simulink model "F500Heli_PIDAttidudeInTheBackLoop"  (R2022b)
settings: Solver=ode3  StartTime=0.0  StopTime=80  FixedStep=0.01  RelTol=1e-3  EnableMultiTasking=on
libraries: simulink_need_slupdate x15, simulink x5
settings Model: Creator=zhi  LastModifiedBy=henrr
settings SolverCC: AlgebraicLoopSolver=TrustRegion
settings DataIOCC: LimitDataPoints=on  SaveFormat=Array  SignalLoggingSaveFormat=ModelDataLogs  ReturnWorkspaceOutputs=off
settings OptimizationCC: ExpressionDepthLimit=2147483647  LifeSpan=inf
settings DebuggingCC: UnderspecifiedInitializationDetection=Classic  MergeDetectMultiDrivingBlocksExec=none  SolverPrmCheckMsg=warning  FcnCallInpInsideContextMsg=warning  UnconnectedInputMsg=warning  UnconnectedOutputMsg=warning  UnconnectedLineMsg=warning  StateNameClashWarn=warning  SFUnexpectedBacktrackingDiag=warning  SFNoUnconditionalDefaultTransitionDiag=warning  SFExecutionAtInitializationDiag=none  SFMachineParentedDataDiag=warning  ArithmeticOperatorsInVariantConditions=warning
settings HardwareCC: ProdBitPerPointer=32  ProdBitPerSizeT=32  ProdBitPerPtrDiffT=32  ProdLargestAtomicFloat=None  ProdIntDivRoundTo=Undefined  ProdEndianess=Unspecified  ProdWordSize=32  ProdHWDeviceType=32-bit Generic
settings ModelReferenceCC: PropagateSignalLabelsOutOfModel=off
settings SFSimCC: SimUseLocalCustomCode=off  SimParseCustomCode=off  CustomCodeUndefinedFunction=UseInterfaceOnly
settings RTWCC: RTWUseLocalCustomCode=off
settings CodeAppCC: StateflowObjectComments=on
settings GRTTargetCC: TargetLangStandard=C89/C90 (ANSI)  CombineOutputUpdateFcns=off  GRTInterface=on
settings ConfigComp: CovMetricSettings=dw  CovSaveCumulativeToWorkspaceVar=on  CovSaveSingleToWorkspaceVar=on  CovExternalEMLEnable=off

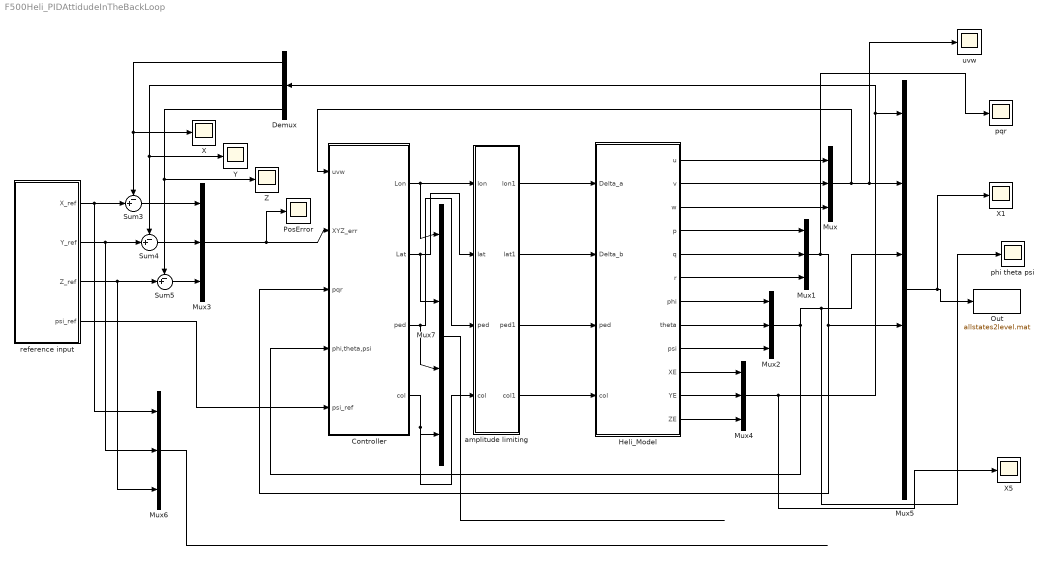
== system F500Heli_PIDAttidudeInTheBackLoop ==
  Controller : Subsystem
  Demux : Demux  Outputs=3
  Heli_Model : Subsystem
  Mux{,1..4,6} (6 alike) : Mux  Inputs=3
  Mux5 : Mux  Inputs=6
  Mux7 : Mux
  Out : ToFile  Filename=allstates2level.mat  MatrixName=AllStates
  PosError : Scope
  Sum3 : Sum  Inputs=-+|
  Sum4 : Sum  Inputs=-+|
  Sum5 : Sum  Inputs=-+|
  X : Scope
  X1 : Scope
  X5 : Scope
  Y : Scope
  Z : Scope
  amplitude limiting : Subsystem
  phi theta psi : Scope
  pqr : Scope
  reference input : Subsystem
  uvw : Scope
  wires:
  Heli_Model/1(u) -> Mux/1
  Heli_Model/2(v) -> Mux/2
  Heli_Model/3(w) -> Mux/3
  Heli_Model/4(p) -> Mux1/1
  Heli_Model/5(q) -> Mux1/2
  Heli_Model/6(r) -> Mux1/3
  Heli_Model/7(phi) -> Mux2/1
  Heli_Model/8(theta) -> Mux2/2
  Heli_Model/9(psi) -> Mux2/3
  Heli_Model/10(XE) -> Mux4/1
  Heli_Model/11(YE) -> Mux4/2
  Heli_Model/12(ZE) -> Mux4/3
  Mux4/1 -> X5/1, Demux/1, Mux5/1
  Mux/1 -> Controller/1(uvw), uvw/1, Mux5/2
  Mux2/1 -> Controller/4(phi,theta,psi), phi theta psi/1, Mux5/3
  Mux1/1 -> pqr/1, Controller/3(pqr), Mux5/4
  Demux/2 -> Sum4/1, Y/1
  Demux/3 -> Sum5/1, Z/1
  reference input/2(Y_ref) -> Sum4/2, Mux6/2
  reference input/3(Z_ref) -> Sum5/2, Mux6/3
  Sum5/1 -> Mux3/3
  Sum4/1 -> Mux3/2
  reference input/1(X_ref) -> Sum3/2, Mux6/1
  Demux/1 -> Sum3/1, X/1
  Sum3/1 -> Mux3/1
  Controller/1(Lon) -> amplitude limiting/1(lon), Mux7/1
  Controller/2(Lat) -> amplitude limiting/2(lat), Mux7/2
  Controller/3(ped) -> amplitude limiting/3(ped), Mux7/3
  Controller/4(col) -> amplitude limiting/4(col), Mux7/4
  amplitude limiting/1(lon1) -> Heli_Model/1(Delta_a)
  amplitude limiting/2(lat1) -> Heli_Model/2(Delta_b)
  amplitude limiting/3(ped1) -> Heli_Model/3(ped)
  amplitude limiting/4(col1) -> Heli_Model/4(col)
  reference input/4(psi_ref) -> Controller/5(psi_ref)
  Mux3/1 -> Controller/2(XYZ_err), PosError/1
  Mux5/1 -> X1/1, Out/1
  Mux7/1 -> ?
  Mux6/1 -> ?

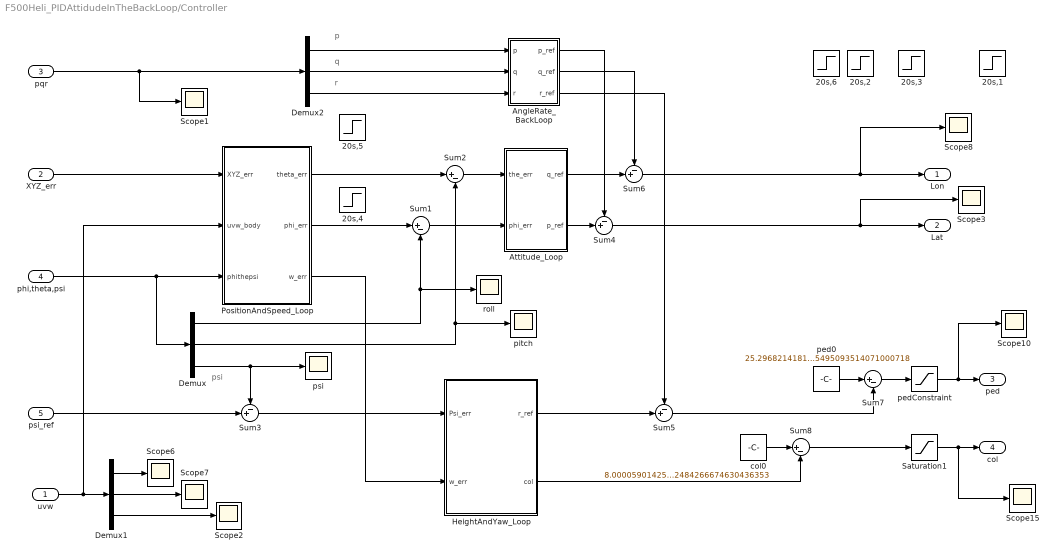
== system F500Heli_PIDAttidudeInTheBackLoop/Controller ==
  note: p
  note: q
  note: r
  note: psi
  uvw : Inport
  XYZ_err : Inport  Port=2
  pqr : Inport  Port=3
  phi,theta,psi : Inport  Port=4
  psi_ref : Inport  Port=5
  20s,1 : Step  Time=0  SampleTime=0
  20s,2 : Step  Time=0  After=0  SampleTime=0
  20s,3 : Step  Time=0  After=25.296753501  SampleTime=0
  20s,4 : Step  Time=0  After=0.2  SampleTime=0
  20s,5 : Step  After=-0.1  SampleTime=0
  20s,6 : Step  Time=0  After=0  SampleTime=0
  AngleRate_BackLoop : Subsystem
  Attitude_Loop : Subsystem
  Demux : Demux  Outputs=3
  Demux1 : Demux  Outputs=3
  Demux2 : Demux  Outputs=3
  HeightAndYaw_Loop : Subsystem
  PositionAndSpeed_Loop : Subsystem
  Saturation1 : Saturate  UpperLimit=12  LowerLimit=0.5
  Scope{1..3,6..8,10,15} (8 alike) : Scope
  Sum{1..2,7..8} (4 alike) : Sum  Inputs=|+-
  Sum{3..6} (4 alike) : Sum  Inputs=-+|
  col0 : Constant  Value=8.0000590142582484266674630436353
  ped0 : Constant  Value=25.296821418115495093514071000718
  pedConstraint : Saturate  UpperLimit=35  LowerLimit=18.7232
  pitch : Scope
  psi : Scope
  roll : Scope
  Lon : Outport
  Lat : Outport  Port=2
  ped : Outport  Port=3
  col : Outport  Port=4
  wires:
  uvw/1 -> Demux1/1, PositionAndSpeed_Loop/2(uvw_body)
  XYZ_err/1 -> PositionAndSpeed_Loop/1(XYZ_err)
  Demux/3 -> Sum3/1, psi/1
  pqr/1 -> Demux2/1, Scope1/1
  Sum3/1 -> HeightAndYaw_Loop/1(Psi_err)
  Demux/1 -> Sum1/2, roll/1
  Demux/2 -> Sum2/2, pitch/1
  Sum2/1 -> Attitude_Loop/1(the_err)
  Sum1/1 -> Attitude_Loop/2(phi_err)
  psi_ref/1 -> Sum3/2
  HeightAndYaw_Loop/1(r_ref) -> Sum5/2
  phi,theta,psi/1 -> Demux/1, PositionAndSpeed_Loop/3(phithepsi)
  Attitude_Loop/2(p_ref) -> Sum4/2
  Attitude_Loop/1(q_ref) -> Sum6/2
  Demux1/3 -> Scope2/1
  Demux1/2 -> Scope7/1
  Demux1/1 -> Scope6/1
  Demux2/2 -> AngleRate_BackLoop/2(q)
  Demux2/1 -> AngleRate_BackLoop/1(p)
  AngleRate_BackLoop/1(p_ref) -> Sum4/1
  AngleRate_BackLoop/2(q_ref) -> Sum6/1
  ped0/1 -> Sum7/1
  Sum7/1 -> pedConstraint/1
  pedConstraint/1 -> ped/1, Scope10/1
  Demux2/3 -> AngleRate_BackLoop/3(r)
  AngleRate_BackLoop/3(r_ref) -> Sum5/1
  col0/1 -> Sum8/1
  Sum8/1 -> Saturation1/1
  Saturation1/1 -> col/1, Scope15/1
  PositionAndSpeed_Loop/3(w_err) -> HeightAndYaw_Loop/2(w_err)
  Sum6/1 -> Lon/1, Scope8/1
  Sum4/1 -> Lat/1, Scope3/1
  Sum5/1 -> Sum7/2
  HeightAndYaw_Loop/2(col) -> Sum8/2
  PositionAndSpeed_Loop/2(phi_err) -> Sum1/1
  PositionAndSpeed_Loop/1(theta_err) -> Sum2/1

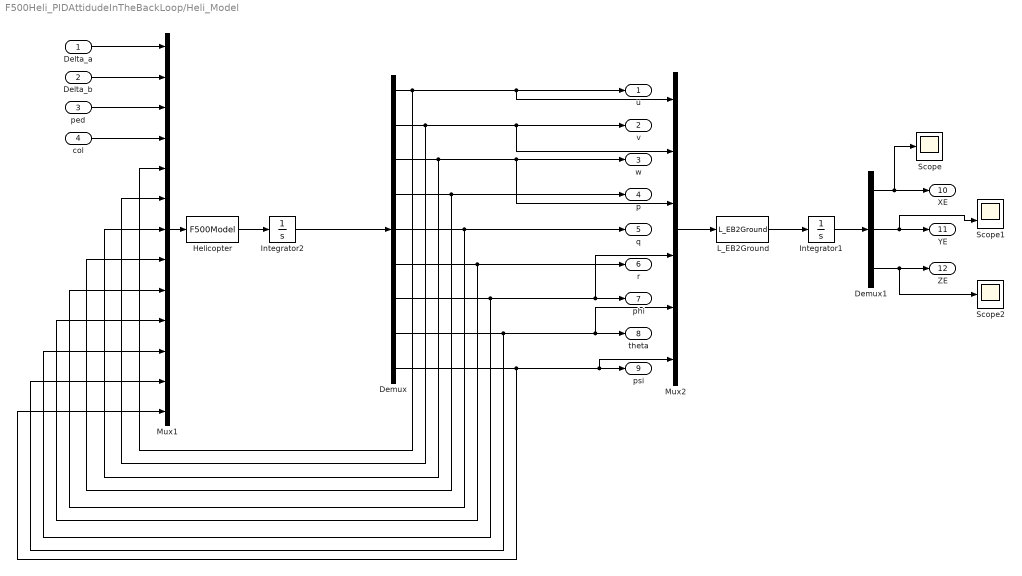
== system F500Heli_PIDAttidudeInTheBackLoop/Heli_Model ==
  Delta_a : Inport
  Delta_b : Inport  Port=2
  ped : Inport  Port=3
  col : Inport  Port=4
  Demux : Demux  Outputs=9
  Demux1 : Demux  Outputs=3
  Helicopter : MATLABFcn  MATLABFcn=F500Model
  Integrator1 : Integrator  InitialCondition=[0 0 0]
  Integrator2 : Integrator  InitialCondition=[0 0 0 0 0 0 0 0 0]
  L_EB2Ground : MATLABFcn  MATLABFcn=L_EB2Ground
  Mux1 : Mux  Inputs=13
  Mux2 : Mux  Inputs=6
  Scope : Scope
  Scope1 : Scope  NumInputPorts=2
  Scope2 : Scope
  u : Outport
  v : Outport  Port=2
  w : Outport  Port=3
  p : Outport  Port=4
  q : Outport  Port=5
  r : Outport  Port=6
  phi : Outport  Port=7
  theta : Outport  Port=8
  psi : Outport  Port=9
  XE : Outport  Port=10
  YE : Outport  Port=11
  ZE : Outport  Port=12
  wires:
  Demux/1 -> Mux1/5, u/1, Mux2/1
  Demux/2 -> Mux1/6, v/1, Mux2/2
  Demux/3 -> Mux1/7, w/1, Mux2/3
  Demux/4 -> Mux1/8, p/1
  Demux/5 -> Mux1/9, q/1
  Demux/6 -> Mux1/10, r/1
  Demux/7 -> Mux1/11, phi/1, Mux2/4
  Demux/8 -> Mux1/12, theta/1, Mux2/5
  Demux/9 -> Mux1/13, psi/1, Mux2/6
  Demux1/1 -> XE/1, Scope/1
  Demux1/2 -> YE/1, Scope1/2
  Demux1/3 -> ZE/1, Scope2/1
  Mux2/1 -> L_EB2Ground/1
  L_EB2Ground/1 -> Integrator1/1
  Integrator1/1 -> Demux1/1
  Mux1/1 -> Helicopter/1
  col/1 -> Mux1/4
  Integrator2/1 -> Demux/1
  ped/1 -> Mux1/3
  Delta_a/1 -> Mux1/1
  Delta_b/1 -> Mux1/2
  Helicopter/1 -> Integrator2/1

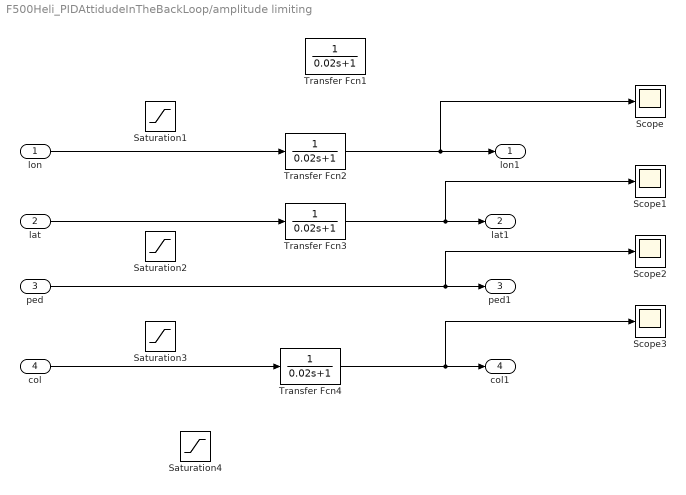
== system F500Heli_PIDAttidudeInTheBackLoop/amplitude limiting ==
  lon : Inport
  lat : Inport  Port=2
  ped : Inport  Port=3
  col : Inport  Port=4
  Saturation1 : Saturate  UpperLimit=0.6  LowerLimit=-0.6
  Saturation2 : Saturate  UpperLimit=0.6  LowerLimit=-0.6
  Saturation3 : Saturate  UpperLimit=0.6  LowerLimit=-0.6
  Saturation4 : Saturate  UpperLimit=10  LowerLimit=-10
  Scope{,1..3} (4 alike) : Scope
  Transfer Fcn{1..4} (4 alike) : TransferFcn  Denominator=[0.02 1]
  lon1 : Outport
  lat1 : Outport  Port=2
  ped1 : Outport  Port=3
  col1 : Outport  Port=4
  wires:
  lon/1 -> Transfer Fcn2/1
  lat/1 -> Transfer Fcn3/1
  col/1 -> Transfer Fcn4/1
  ped/1 -> ped1/1, Scope2/1
  Transfer Fcn2/1 -> lon1/1, Scope/1
  Transfer Fcn3/1 -> lat1/1, Scope1/1
  Transfer Fcn4/1 -> col1/1, Scope3/1

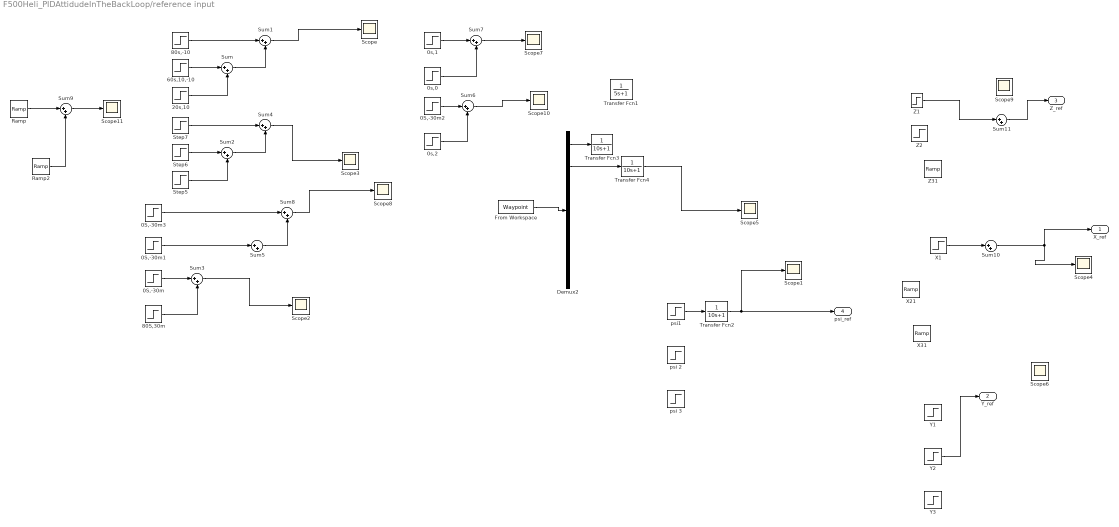
== system F500Heli_PIDAttidudeInTheBackLoop/reference input ==
  0S,-30m : Step  Time=70  After=-3  SampleTime=0
  0S,-30m1 : Step  Time=60  Before=10  After=5  SampleTime=0
  0S,-30m2 : Step  Time=10  After=10  SampleTime=0
  0S,-30m3 : Step  Time=70  Before=5  After=0  SampleTime=0
  0s,0 : Step  Time=10  After=0  SampleTime=0
  0s,1 : Step  Time=0  After=5  SampleTime=0
  0s,2 : Step  Time=0  After=5  SampleTime=0
  20s,10 : Step  Time=20  After=5  SampleTime=0
  60s,10,-10 : Step  Time=30  Before=5  After=-5  SampleTime=0
  80S,30m : Step  Time=10  After=3  SampleTime=0
  80s,-10 : Step  Time=40  Before=-5  After=0  SampleTime=0
  Demux2 : Demux  Outputs=7
  From Workspace : FromWorkspace  VariableName=Waypoint
  Ramp : simulink/Sources/Ramp  slope=1  start=0  InitialOutput=0
  Ramp2 : simulink/Sources/Ramp  slope=-1  start=20  InitialOutput=0
  Scope{,1..11} (12 alike) : Scope
  Step5 : Step  Time=40  After=5  SampleTime=0
  Step6 : Step  Time=50  Before=5  After=-5  SampleTime=0
  Step7 : Step  Time=60  Before=-5  After=0  SampleTime=0
  Sum{,1..11} (12 alike) : Sum  Inputs=|++
  Transfer Fcn1 : TransferFcn  Denominator=[5 1]
  Transfer Fcn2 : TransferFcn  Denominator=[10 1]
  Transfer Fcn3 : TransferFcn  Denominator=[10 1]
  Transfer Fcn4 : TransferFcn  Denominator=[10 1]
  X1 : Step  Time=0  After=20  SampleTime=0
  X21 : simulink/Sources/Ramp  slope=1  start=15  InitialOutput=0
  X31 : simulink/Sources/Ramp  slope=1  start=20  InitialOutput=0
  Y1 : Step  Time=0  After=5  SampleTime=0
  Y2 : Step  Time=0  After=10  SampleTime=0
  Y3 : Step  Time=0  After=5  SampleTime=0
  Z1 : Step  Time=0  After=20  SampleTime=0
  Z2 : Step  Time=10  After=10  SampleTime=0
  Z31 : simulink/Sources/Ramp  slope=1  start=0  InitialOutput=0
  psi 2 : Step  Time=5  After=0.2  SampleTime=0
  psi 3 : Step  Time=0  After=0  SampleTime=0
  psi1 : Step  Time=0  After=0  SampleTime=0
  X_ref : Outport
  Y_ref : Outport  Port=2
  Z_ref : Outport  Port=3
  psi_ref : Outport  Port=4
  wires:
  20s,10/1 -> Sum/2
  60s,10,-10/1 -> Sum/1
  80s,-10/1 -> Sum1/1
  Sum/1 -> Sum1/2
  Sum1/1 -> Scope/1
  Step5/1 -> Sum2/2
  Step6/1 -> Sum2/1
  Step7/1 -> Sum4/1
  Sum2/1 -> Sum4/2
  Sum4/1 -> Scope3/1
  0S,-30m/1 -> Sum3/1
  80S,30m/1 -> Sum3/2
  0S,-30m1/1 -> Sum5/1
  0S,-30m2/1 -> Sum6/1
  0s,2/1 -> Sum6/2
  0s,1/1 -> Sum7/1
  0s,0/1 -> Sum7/2
  Sum8/1 -> Scope8/1
  Sum5/1 -> Sum8/2
  0S,-30m3/1 -> Sum8/1
  Sum3/1 -> Scope2/1
  From Workspace/1 -> Demux2/1
  Demux2/1 -> Transfer Fcn3/1
  Demux2/2 -> Transfer Fcn4/1
  Transfer Fcn2/1 -> psi_ref/1, Scope1/1
  Transfer Fcn4/1 -> Scope5/1
  Sum7/1 -> Scope7/1
  Sum6/1 -> Scope10/1
  Ramp/1 -> Sum9/1
  Sum9/1 -> Scope11/1
  Ramp2/1 -> Sum9/2
  Sum10/1 -> Scope4/1, X_ref/1
  Sum11/1 -> Z_ref/1
  Y2/1 -> Y_ref/1
  psi1/1 -> Transfer Fcn2/1
  Z1/1 -> Sum11/1
  X1/1 -> Sum10/1

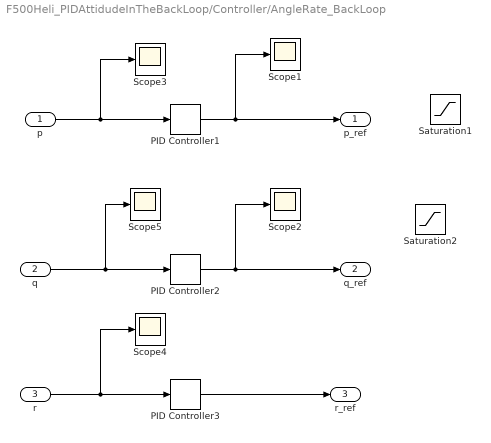
== system F500Heli_PIDAttidudeInTheBackLoop/Controller/AngleRate_BackLoop ==
  p : Inport
  q : Inport  Port=2
  r : Inport  Port=3
  PID Controller1 : simulink_need_slupdate/PID Controller  P=5  I=0  D=0
  PID Controller2 : simulink_need_slupdate/PID Controller  P=5  I=0  D=0
  PID Controller3 : simulink_need_slupdate/PID Controller  P=10  I=0  D=0
  Saturation1 : Saturate  UpperLimit=10  LowerLimit=-10
  Saturation2 : Saturate  UpperLimit=10  LowerLimit=-10
  Scope{1..5} (5 alike) : Scope
  p_ref : Outport
  q_ref : Outport  Port=2
  r_ref : Outport  Port=3
  wires:
  PID Controller1/1 -> Scope1/1, p_ref/1
  p/1 -> PID Controller1/1, Scope3/1
  PID Controller2/1 -> Scope2/1, q_ref/1
  q/1 -> PID Controller2/1, Scope5/1
  r/1 -> PID Controller3/1, Scope4/1
  PID Controller3/1 -> r_ref/1

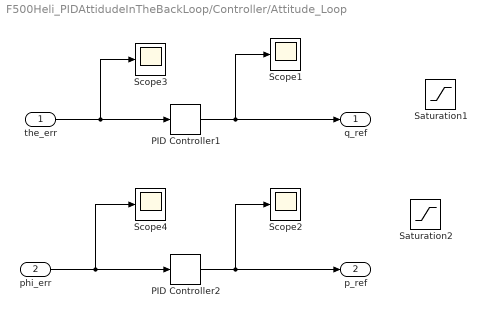
== system F500Heli_PIDAttidudeInTheBackLoop/Controller/Attitude_Loop ==
  the_err : Inport
  phi_err : Inport  Port=2
  PID Controller1 : simulink_need_slupdate/PID Controller  P=20  I=5  D=0
  PID Controller2 : simulink_need_slupdate/PID Controller  P=18  I=5  D=0
  Saturation1 : Saturate  UpperLimit=3  LowerLimit=-3
  Saturation2 : Saturate  UpperLimit=3  LowerLimit=-3
  Scope{1..4} (4 alike) : Scope
  q_ref : Outport
  p_ref : Outport  Port=2
  wires:
  PID Controller1/1 -> Scope1/1, q_ref/1
  the_err/1 -> PID Controller1/1, Scope3/1
  PID Controller2/1 -> Scope2/1, p_ref/1
  phi_err/1 -> PID Controller2/1, Scope4/1

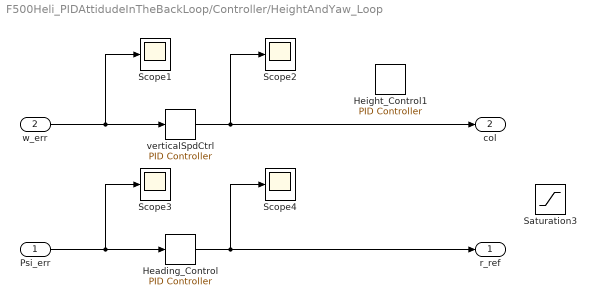
== system F500Heli_PIDAttidudeInTheBackLoop/Controller/HeightAndYaw_Loop ==
  Psi_err : Inport
  w_err : Inport  Port=2
  Heading_Control : simulink_need_slupdate/PID Controller  P=5  I=0  D=0.5
  Height_Control1 : simulink_need_slupdate/PID Controller  P=1  I=0.01  D=1.4
  Saturation3 : Saturate  UpperLimit=36  LowerLimit=18.7232
  Scope{1..4} (4 alike) : Scope
  verticalSpdCtrl : simulink_need_slupdate/PID Controller  P=5  I=0  D=0
  r_ref : Outport
  col : Outport  Port=2
  wires:
  w_err/1 -> verticalSpdCtrl/1, Scope1/1
  verticalSpdCtrl/1 -> Scope2/1, col/1
  Heading_Control/1 -> Scope4/1, r_ref/1
  Psi_err/1 -> Heading_Control/1, Scope3/1

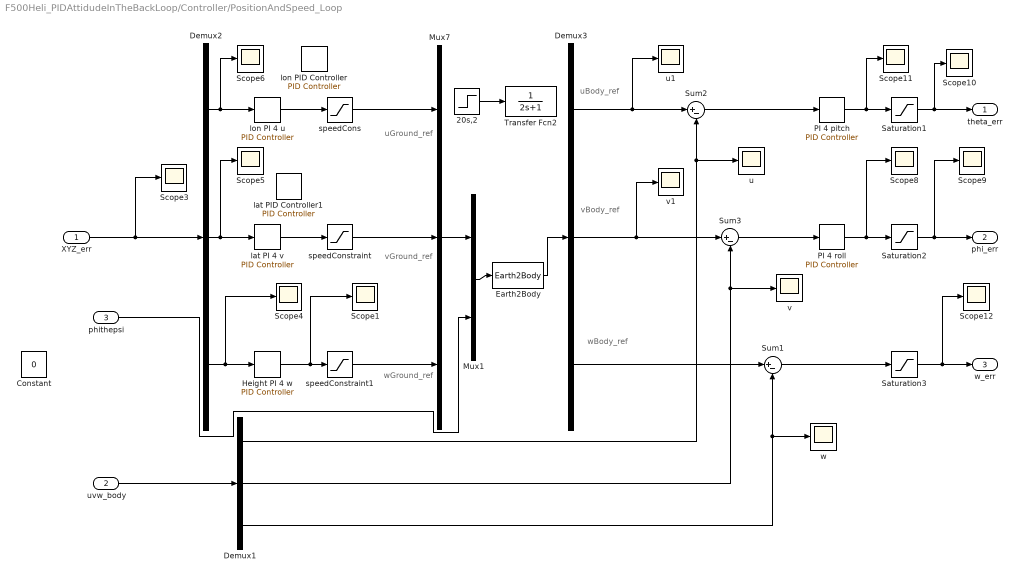
== system F500Heli_PIDAttidudeInTheBackLoop/Controller/PositionAndSpeed_Loop ==
  note: uGround_ref
  note: vGround_ref
  note: wGround_ref
  note: uBody_ref
  note: vBody_ref
  note: wBody_ref
  XYZ_err : Inport
  uvw_body : Inport  Port=2
  phithepsi : Inport  Port=3
  20s,2 : Step  Time=10  After=5  SampleTime=0
  Constant : Constant  Value=0
  Demux1 : Demux  Outputs=3
  Demux2 : Demux  Outputs=3
  Demux3 : Demux  Outputs=3
  Earth2Body : MATLABFcn  MATLABFcn=Earth2Body  OutputDimensions=3
  Height PI 4 w : simulink_need_slupdate/PID Controller  P=1  I=0.002  D=0
  Mux1 : Mux  Inputs=2
  Mux7 : Mux  Inputs=3
  PI 4 pitch : simulink_need_slupdate/PID Controller  P=-0.7  I=0.0001  D=0
  PI 4 roll : simulink_need_slupdate/PID Controller  P=0.7  I=0.0001  D=0
  Saturation1 : Saturate  UpperLimit=0.1745  LowerLimit=-0.5236
  Saturation2 : Saturate  UpperLimit=0.6109  LowerLimit=-0.6109
  Saturation3 : Saturate  UpperLimit=0.6109  LowerLimit=-0.6109
  Scope{1,3..6,8..12} (10 alike) : Scope
  Sum1 : Sum  Inputs=|+-
  Sum2 : Sum  Inputs=|+-
  Sum3 : Sum  Inputs=|+-
  Transfer Fcn2 : TransferFcn  Denominator=[2 1]
  lat PI 4 v : simulink_need_slupdate/PID Controller  P=1  I=0.0001  D=0
  lat PID Controller1 : simulink_need_slupdate/PID Controller  P=1  I=0.0001  D=2
  lon PI 4 u : simulink_need_slupdate/PID Controller  P=1  I=0.0001  D=0
  lon PID Controller : simulink_need_slupdate/PID Controller  P=-1  I=0.0001  D=-2
  speedCons : Saturate  UpperLimit=10  LowerLimit=-10
  speedConstraint : Saturate  UpperLimit=2  LowerLimit=-2
  speedConstraint1 : Saturate  UpperLimit=3  LowerLimit=-3
  u : Scope
  u1 : Scope
  v : Scope
  v1 : Scope
  w : Scope
  theta_err : Outport
  phi_err : Outport  Port=2
  w_err : Outport  Port=3
  wires:
  Demux2/1 -> lon PI 4 u/1, Scope6/1
  lon PI 4 u/1 -> speedCons/1
  lat PI 4 v/1 -> speedConstraint/1
  Demux2/2 -> lat PI 4 v/1, Scope5/1
  Demux2/3 -> Height PI 4 w/1, Scope4/1
  XYZ_err/1 -> Demux2/1, Scope3/1
  Height PI 4 w/1 -> speedConstraint1/1, Scope1/1
  uvw_body/1 -> Demux1/1
  speedCons/1 -> Mux7/1
  speedConstraint/1 -> Mux7/2
  speedConstraint1/1 -> Mux7/3
  Earth2Body/1 -> Demux3/1
  Demux1/1 -> Sum2/2, u/1
  Demux1/2 -> Sum3/2, v/1
  Demux1/3 -> Sum1/2, w/1
  Sum2/1 -> PI 4 pitch/1
  PI 4 pitch/1 -> Saturation1/1, Scope11/1
  Saturation1/1 -> theta_err/1, Scope10/1
  Sum3/1 -> PI 4 roll/1
  Sum1/1 -> Saturation3/1
  Saturation3/1 -> w_err/1, Scope12/1
  PI 4 roll/1 -> Saturation2/1, Scope8/1
  Saturation2/1 -> phi_err/1, Scope9/1
  Mux7/1 -> Mux1/1
  phithepsi/1 -> Mux1/2
  Mux1/1 -> Earth2Body/1
  20s,2/1 -> Transfer Fcn2/1
  Demux3/3 -> Sum1/1
  Demux3/2 -> Sum3/1, v1/1
  Demux3/1 -> Sum2/1, u1/1
